simulink model "Week2_Problem4"  (R2020b)
settings: Solver=VariableStepAuto  StartTime=0.0  StopTime=0.2  RelTol=1e-3
settings Model: DataDictionary=Problem4_data.sldd  Creator=ASUS  LastModifiedBy=ASUS
settings SolverCC: AlgebraicLoopSolver=LineSearch
settings DebuggingCC: ModelReferenceExtraNoncontSigs=none

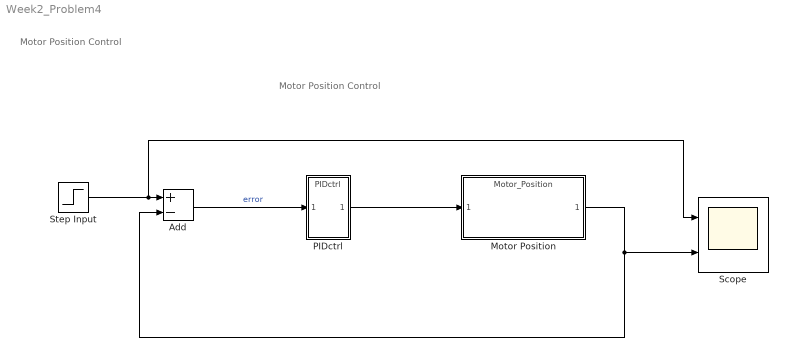
== system Week2_Problem4 ==
  note: Motor Position Control
  note: Motor Position Control
  Add : Sum  Inputs=+-
  "Motor Position " : ModelReference  ModelNameDialog=Motor_Position  SimulationMode=Normal  ModelReferenceVersion=1.3
  PIDctrl : ModelReference  ModelNameDialog=PIDctrl  SimulationMode=Normal  ModelReferenceVersion=1.9
  Scope : Scope  NumInputPorts=2
  Step Input : Step  Time=0  SampleTime=0
  wires:
  Step Input/1 -> Scope/1, Add/1
  "Motor Position "/1 -> Add/2, Scope/2
  Add/1 -> PIDctrl/1  "error"
  PIDctrl/1 -> "Motor Position "/1
